simulink model "Test_N2"  (R2022a)
settings: Solver=ode3  StartTime=0.0  StopTime=inf  FixedStep=0.05  RelTol=1e-3
libraries: Utilities x5, EcBlockToolbox x1

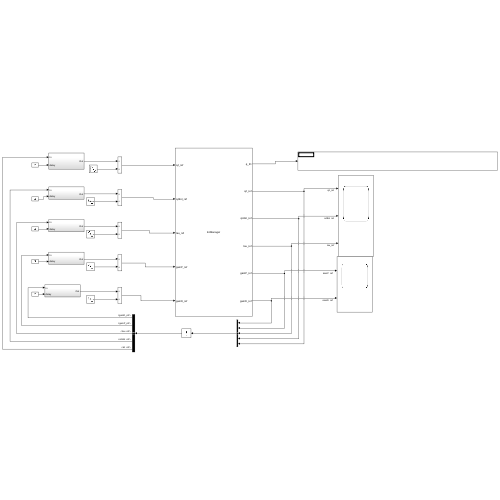
[thumbnail: Simulink's stored preview of the top-level diagram]
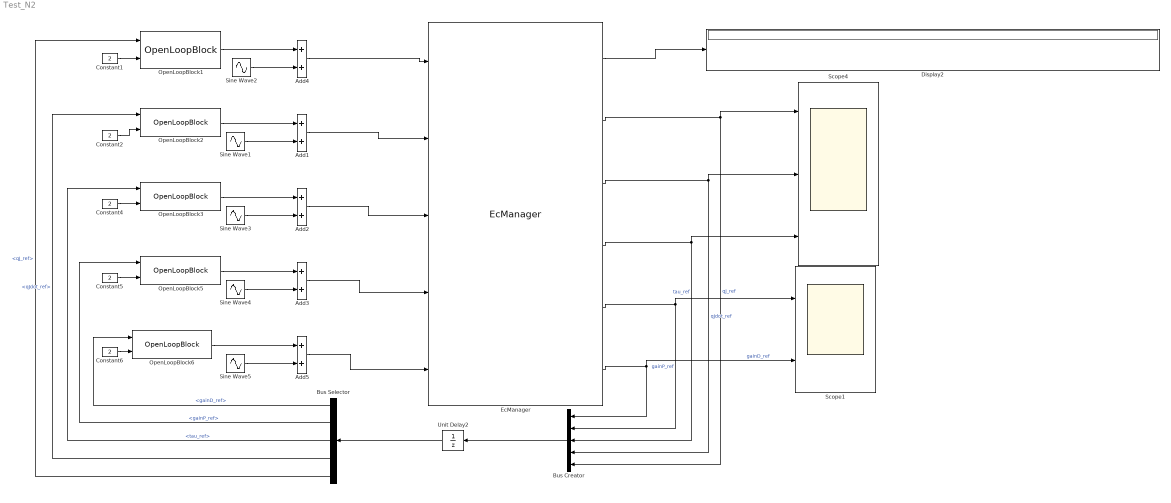
== system Test_N2 ==
  Add{1..5} (5 alike) : Sum
  Bus Creator : BusCreator  Inputs=5
  Bus Selector : BusSelector  OutputSignals=gainD_ref,gainP_ref,tau_ref,qJdot_ref,qJ_ref
  Constant{1..2,4..6} (5 alike) : Constant  Value=2
  Display2 : Display
  EcManager : EcBlockToolbox/EcManager  ReadingsList={'q_ID', 'qJ_ref', 'qJdot_ref', 'tau_ref', 'gainP_ref', 'gainD_ref'}  ReferencesList={'qJ_ref', 'qJdot_ref', 'tau_ref', 'gainP_ref', 'gainD_ref'}  ImuList={}
  OpenLoopBlock{1..3,5..6} (5 alike) : Utilities/OpenLoopBlock  SystemSampleTime=-1  VariantActivationTime=update diagram  Latency=0  AutoFrameSizeCalculation=off
  Scope1 : Scope  NumInputPorts=2
  Scope4 : Scope  NumInputPorts=3
  Sine Wave1 : Sin  Amplitude=10  SampleTime=0
  Sine Wave2 : Sin  Amplitude=5  SampleTime=0
  Sine Wave3 : Sin  Amplitude=300  SampleTime=0
  Sine Wave4 : Sin  Amplitude=200  SampleTime=0
  Sine Wave5 : Sin  Amplitude=10  SampleTime=0
  Unit Delay2 : UnitDelay  SampleTime=-1  HasFrameUpgradeWarning=on
  wires:
  EcManager/6 -> Scope1/2, Bus Creator/1  "gainD_ref"
  Sine Wave2/1 -> Add4/2
  EcManager/4 -> Scope4/3, Bus Creator/3  "tau_ref"
  EcManager/1 -> Display2/1
  EcManager/5 -> Scope1/1, Bus Creator/2  "gainP_ref"
  Sine Wave1/1 -> Add1/2
  EcManager/2 -> Scope4/1, Bus Creator/5  "qJ_ref"
  Sine Wave3/1 -> Add2/2
  EcManager/3 -> Scope4/2, Bus Creator/4  "qJdot_ref"
  Add4/1 -> EcManager/1
  Add1/1 -> EcManager/2
  Add2/1 -> EcManager/3
  Add3/1 -> EcManager/4
  Sine Wave4/1 -> Add3/2
  Add5/1 -> EcManager/5
  Sine Wave5/1 -> Add5/2
  Bus Creator/1 -> Unit Delay2/1
  Bus Selector/1 -> OpenLoopBlock6/1  "<gainD_ref>"
  Bus Selector/2 -> OpenLoopBlock5/1  "<gainP_ref>"
  Unit Delay2/1 -> Bus Selector/1
  Bus Selector/3 -> OpenLoopBlock3/1  "<tau_ref>"
  Bus Selector/4 -> OpenLoopBlock2/1  "<qJdot_ref>"
  Bus Selector/5 -> OpenLoopBlock1/1  "<qJ_ref>"
  OpenLoopBlock1/1 -> Add4/1
  Constant1/1 -> OpenLoopBlock1/2
  Constant2/1 -> OpenLoopBlock2/2
  OpenLoopBlock2/1 -> Add1/1
  Constant4/1 -> OpenLoopBlock3/2
  OpenLoopBlock3/1 -> Add2/1
  OpenLoopBlock5/1 -> Add3/1
  Constant5/1 -> OpenLoopBlock5/2
  OpenLoopBlock6/1 -> Add5/1
  Constant6/1 -> OpenLoopBlock6/2
